simulink model "simpleTreeDiff"  (R2023b)
settings: Solver=VariableStepAuto  StartTime=0.0  StopTime=10.0  RelTol=1e-3
settings Model: Creator=neham  LastModifiedBy=neham

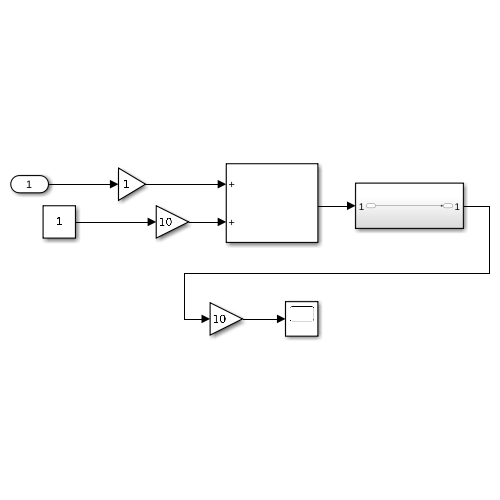
[thumbnail: Simulink's stored preview of the top-level diagram]
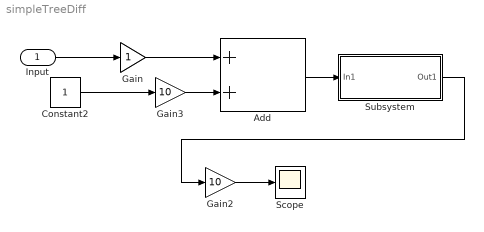
== system simpleTreeDiff ==
  Input : Inport
  Add : Sum
  Constant2 : Constant
  Gain : Gain
  Gain2 : Gain  Gain=10
  Gain3 : Gain  Gain=10
  Scope : Scope
  Subsystem : Subsystem
  wires:
  Input/1 -> Gain/1
  Gain/1 -> Add/1
  Subsystem/1(Out1) -> Gain2/1
  Constant2/1 -> Gain3/1
  Gain3/1 -> Add/2
  Add/1 -> Subsystem/1(In1)
  Gain2/1 -> Scope/1

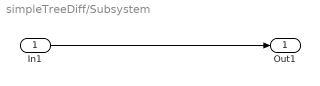
== system simpleTreeDiff/Subsystem ==
  In1 : Inport
  Out1 : Outport
  wires:
  In1/1 -> Out1/1
